simulink model "sfbuilder_multiport"  (Simulink 7.6)
settings: Solver=ode1  SolverMode=SingleTasking  StartTime=0.0  StopTime=10.0  RelTol=1e-3
settings Model: Creator=The MathWorks Inc.  ExtModeAutoUpdateStatusClock=off
settings DataIOCC: SignalLoggingName=sigsOut
settings OptimizationCC: BooleanDataType=off
settings DebuggingCC: SaveWithParameterizedLinksMsg=none  SignalResolutionControl=TryResolveAllWithWarning  SolverPrmCheckMsg=none  MultiTaskDSMMsg=warning  MultiTaskCondExecSysMsg=none
settings HardwareCC: TargetUnknown=on
settings RTWCC: IncludeERTFirstTime=on

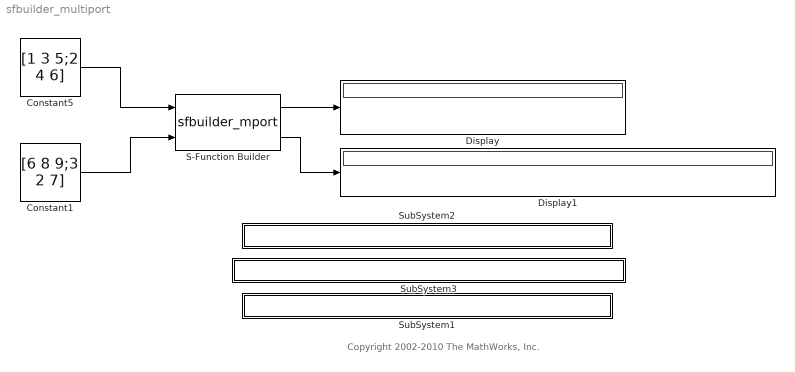
== system sfbuilder_multiport ==
  note: Copyright 2002-2010 The MathWorks, Inc.
  Constant1 : Constant  Value=[6 8 9;3 2 7]  VectorParams1D=off  OutDataTypeStr=int32
  Constant5 : Constant  Value=[1 3 5;2 4 6]  VectorParams1D=off  OutDataTypeStr=single
  Display : Display
  Display1 : Display
  S-Function Builder : S-Function  FunctionName=sfbuilder_mport  SFunctionModules=sfbuilder_mport_wrapper  WizardData=DataTag0  EnableBusSupport=off  mask(S-Function Builder){}
      mask init:
      | val = [[.9  0.75 0.75 1 1 .9 .9 1]',[1 1 0.75 0.75 .9 .9 1 .9]'];
      | sys = get_param(gcb,'FunctionName');
      settings: CopyFcn=set_param(gcb,'LinkStatus','none')  OpenFcn=sfunctionwizard(gcbh)
      mask Display:
      | plot(val(:,1),val(:,2))
      | disp(sys)
      | port_label('input',1,'in1')
      | port_label('input',2,'in2')
      | port_label('output',1,'out1')
      | port_label('output',2,'out2')
  SubSystem1 : Subsystem  mask{filename=sfbuilder_mport.tlc}
      mask init:
      | x=sfundemo_maskdisp;
      settings: AttributesFormatString=\n  OpenFcn=sfundemo_openfcn
      mask Display: disp(x);
  SubSystem2 : Subsystem  mask{filename=sfbuilder_mport.c}
      mask init:
      | x=sfundemo_maskdisp;
      settings: AttributesFormatString=\n  OpenFcn=sfundemo_openfcn
      mask Display: disp(x);
  SubSystem3 : Subsystem  mask{filename=sfbuilder_mport_wrapper.c}
      mask init:
      | x=sfundemo_maskdisp;
      settings: AttributesFormatString=\n  OpenFcn=sfundemo_openfcn
      mask Display: disp(x);
  wires:
  Constant1/1 -> S-Function Builder/2
  Constant5/1 -> S-Function Builder/1
  S-Function Builder/1 -> Display/1
  S-Function Builder/2 -> Display1/1

== system sfbuilder_multiport/SubSystem1 ==

== system sfbuilder_multiport/SubSystem2 ==

== system sfbuilder_multiport/SubSystem3 ==
